simulink model "ex1s"  (R2020a)
settings: Solver=VariableStepAuto  StartTime=0.0  StopTime=10.0  RelTol=1e-3
values from neighbouring files (symbols this model uses):
  den_Gd = poly(r)    [ex1.m]
  num_Gd = [120 120]    [ex1.m]
libraries: simulink x4

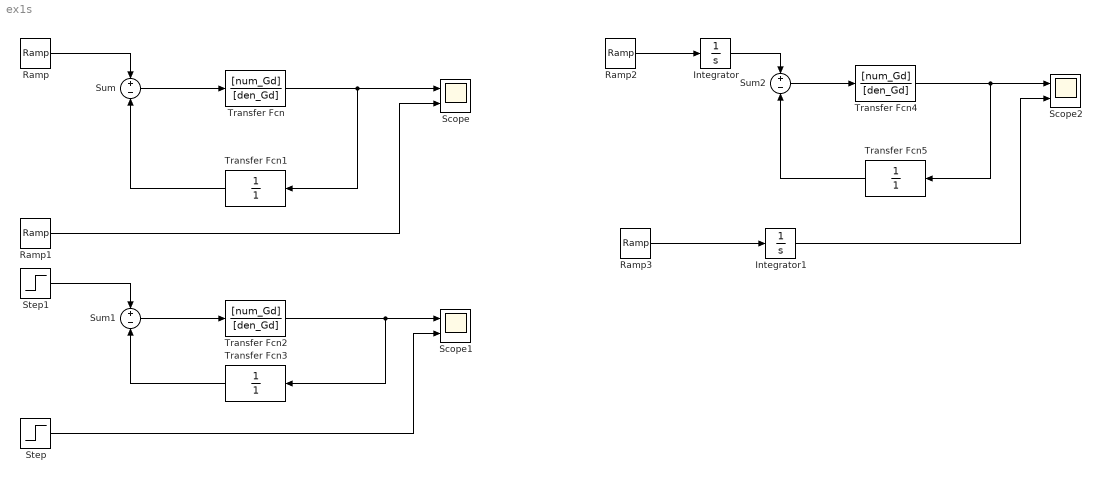
== system ex1s ==
  Integrator : Integrator
  Integrator1 : Integrator
  Ramp{,1..3} (4 alike) : simulink/Sources/Ramp  slope=1  start=0  InitialOutput=0
  Scope : Scope  NumInputPorts=2
  Scope1 : Scope  NumInputPorts=2
  Scope2 : Scope  NumInputPorts=2
  Step : Step  SampleTime=0
  Step1 : Step  SampleTime=0
  Sum : Sum  Inputs=+-
  Sum1 : Sum  Inputs=+-
  Sum2 : Sum  Inputs=+-
  Transfer Fcn : TransferFcn  Numerator=[num_Gd]  Denominator=[den_Gd]
  Transfer Fcn1 : TransferFcn  Denominator=[1]
  Transfer Fcn2 : TransferFcn  Numerator=[num_Gd]  Denominator=[den_Gd]
  Transfer Fcn3 : TransferFcn  Denominator=[1]
  Transfer Fcn4 : TransferFcn  Numerator=[num_Gd]  Denominator=[den_Gd]
  Transfer Fcn5 : TransferFcn  Denominator=[1]
  wires:
  Sum/1 -> Transfer Fcn/1
  Transfer Fcn/1 -> Transfer Fcn1/1, Scope/1
  Transfer Fcn1/1 -> Sum/2
  Ramp/1 -> Sum/1
  Ramp1/1 -> Scope/2
  Step1/1 -> Sum1/1
  Sum1/1 -> Transfer Fcn2/1
  Transfer Fcn2/1 -> Transfer Fcn3/1, Scope1/1
  Transfer Fcn3/1 -> Sum1/2
  Step/1 -> Scope1/2
  Sum2/1 -> Transfer Fcn4/1
  Transfer Fcn4/1 -> Transfer Fcn5/1, Scope2/1
  Transfer Fcn5/1 -> Sum2/2
  Ramp2/1 -> Integrator/1
  Integrator/1 -> Sum2/1
  Ramp3/1 -> Integrator1/1
  Integrator1/1 -> Scope2/2
